simulink model "ysw9_7sim"  (Simulink 8.3)
settings: Solver=ode45  SolverMode=SingleTasking  StartTime=0.0  StopTime=10  FixedStep=0.001  RelTol=1e-3
settings Model: Creator=ljk  LastModifiedBy=ii  ExtModeTrigMode=oneshot  ExtModeArmWhenConnect=off
settings DataIOCC: LimitDataPoints=off
settings OptimizationCC: BlockReduction=off  BooleanDataType=off  ExpressionDepthLimit=2147483647
settings DebuggingCC: SaveWithParameterizedLinksMsg=none  SignalResolutionControl=TryResolveAllWithWarning  SolverPrmCheckMsg=none  MultiTaskDSMMsg=warning  MultiTaskCondExecSysMsg=none  FcnCallInpInsideContextMsg=UseLocalSettings
settings HardwareCC: TargetUnknown=on
settings RTWCC: IncludeERTFirstTime=on

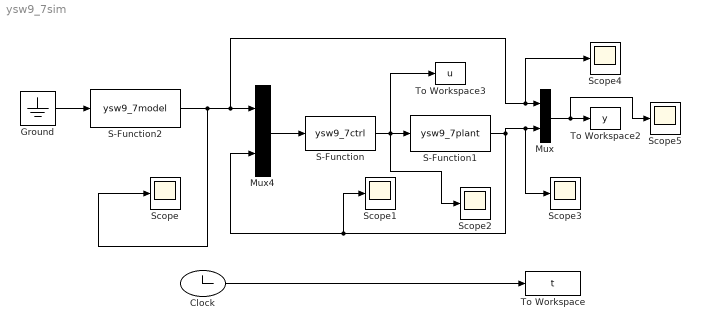
== system ysw9_7sim ==
  Clock : Clock
  Ground : Ground
  Mux : Mux  Inputs=2
  Mux4 : Mux  Inputs=2
  S-Function : S-Function  FunctionName=ysw9_7ctrl  EnableBusSupport=off
  S-Function1 : S-Function  FunctionName=ysw9_7plant  EnableBusSupport=off
  S-Function2 : S-Function  FunctionName=ysw9_7model  EnableBusSupport=off
  Scope{,1..5} (6 alike) : Scope
      Scope2 settings: SaveName=ScopeData2
      Scope3 settings: SaveName=ScopeData3
      Scope4 settings: SaveName=ScopeData4
      Scope5 settings: SaveName=ScopeData5
  To Workspace : ToWorkspace  VariableName=t  SampleTime=-1
  To Workspace2 : ToWorkspace  VariableName=y  SampleTime=-1
  To Workspace3 : ToWorkspace  VariableName=u  SampleTime=-1
  wires:
  Mux4/1 -> S-Function/1
  S-Function1/1 -> Scope1/1, Mux4/2, Scope3/1, Mux/2
  S-Function2/1 -> Scope/1, Scope4/1, Mux/1, Mux4/1
  Ground/1 -> S-Function2/1
  Clock/1 -> To Workspace/1
  Mux/1 -> Scope5/1, To Workspace2/1
  S-Function/1 -> Scope2/1, S-Function1/1, To Workspace3/1
